simulink model "Charging"  (R2021a)
settings: Solver=VariableStepAuto  StartTime=0.0  StopTime=6000  RelTol=1e-3
undefined symbols (not defined in the file or in its folder): Ion, Lithium
libraries: spsBreakerLib x2, spsStairGeneratorLib x1, spsBatteryLib x1, simulink x1, spsControlledCurrentSourceLib x1, spsControlledVoltageSourceLib x1, spsVoltageMeasurementLib x1, spspowerguiLib x1
settings Model: Creator=Samiran  LastModifiedBy=Samiran

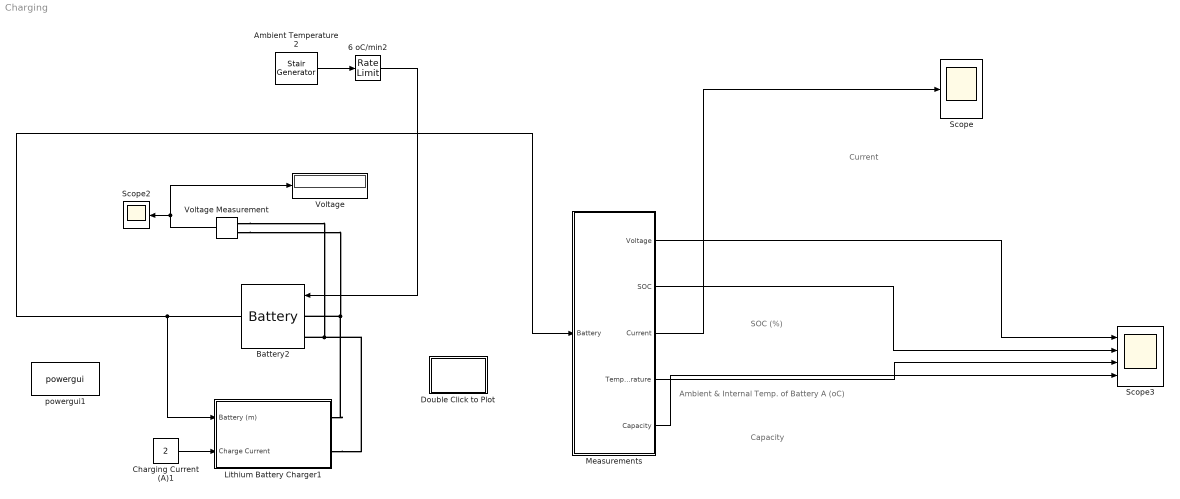
== system Charging ==
  note: Current
  note: Capacity
  note: SOC (%)
  note: Ambient & Internal Temp. of Battery A (oC)
  6 oC/min2 : RateLimiter  RisingSlewLimit=0.5  FallingSlewLimit=-0.5  SampleTimeMode=inherited
  Ambient Temperature2 : spsStairGeneratorLib/Stair Generator  t="[0, 500, 1000 1500  2000 2500 3000]"  e="[25, 0, -20  0  20, 50 20]"  Ts=0
  Battery2 : spsBatteryLib/Battery  BatType=Lithium-Ion  ShowTempParam=on  ThermalPreset="3.6V  3.6Ah  (LiNiO2)"  ShowAgeParam=on  NomV=3.1  NomQ=3.6  SOC=50  Batt_Tr=30  PresetModel=off  MaxQ=3.2  MinV=2.325  FullV=3.75  Dis_rate=0.72  R=0.00889  Normal_OP=2.8  expZone="[3.5         0.5]"  current=[6.5 13 32.5]  Units=Time  Tci=20  NomT=20  T2=0  MaxQ2=2.7  FullV2=3.5  Normal_OP2=2.94  expZone2="[3.25         0.5]"  Rca=0.6  ti=1000  Dp=0  Neq0=0  Tsim=1e6  Ta1=25  Qeol=5.4*0.9  Reol=0.013333*1.2  Char_age=[2.3478, 3]  Dis_age=[2.3478, 10]  N1=1500  N2=10500  N3=1000  N4=1400  Ta2=45  N5=950
  Charging Current (A)1 : Constant  Value=2
  Double Click to Plot : Subsystem
      settings: OpenFcn=LithiumBatteryChargingPlot
      mask Display: fprintf('Battery \n Charge Plot')
  Lithium Battery Charger1 : Subsystem  mask(Lithium Battery Charger){CV=4.2}
      mask prompts: CV "Saturation Charge Constant Voltage (V)"
      mask help:
      | Lithium Battery Charger Block Developed By Rodney Tan (PhD)
      | Version 1.00 (Aug 2019)
      |
      | This charger charge Lithium-Ion battery in two stages
      | This charger takes in charge current (A) from the input in (CC) Constant Current charging stage and switch to Saturation Charge (CV) Constant Voltage charging stage when the battery reaches the set constant voltage.
  Measurements : Subsystem
  Scope : Scope
  Scope2 : Scope
  Scope3 : Scope  NumInputPorts=4
  Voltage : Display
  Voltage Measurement : spsVoltageMeasurementLib/Voltage Measurement  PhasorSimulation=off  OutputType=Complex  PSBequivalent=0
  powergui1 : spspowerguiLib/powergui  Priority=1  SimulationMode=Continuous  SampleTime=50e-6  frequency=60  Iterations=50  frequencyindice=0  Pbase=100e6  ErrMax=1e-4  UnitsV=kV  UnitsW=MW  buscounter=0  FunctionMessages=off  echomessages=off  EnableUseOfTLC=off  CurrentSourceSwitches=off  DisableSnubberDevices=off  DisableRonSwitches=off  DisableVfSwitches=off  DisplayEquations=off  AutomaticDiscreteSolvers=off  SolverType=Tustin/Backward Euler (TBE)  Interpol=off  ExternalGateDelay=off  methode=off  Ts=100  x0status=blocks  SPID=on  SwTol=0  HookPort=off  NonlinearTolerance=1e-4  nMaxIteration=100  ContinueOnMaxIteration=off  RestoreLinks=warning  ResistiveCurrentMeasurement=off  Frange=[0:2:500]  Ylog=off  Xlog=on  ShowGrid=off  save=off  variable=ZData  structure=0  ZoomFFT=off  StartTime=0.0  cycles=1  DisplayStyle=1  fundamental=60  FreqAxis=off  MaxFrequency=1000  frequencyindicesteady=1  RmsSteady=1  display=off
  wires:
  Battery2/1 -> Lithium Battery Charger1/1(Battery (m)), Measurements/1("Battery ")
  6 oC/min2/1 -> Battery2/1
  Ambient Temperature2/1 -> 6 oC/min2/1
  Voltage Measurement/1 -> Voltage/1, Scope2/1
  Measurements/2(SOC) -> Scope3/2
  Charging Current (A)1/1 -> Lithium Battery Charger1/2(Charge Current)
  Measurements/4(Temperature) -> Scope3/3
  Measurements/5(Capacity) -> Scope3/4
  Measurements/1(Voltage) -> Scope3/1
  Measurements/3(Current) -> Scope/1
  connections:
  Voltage Measurement/LConn1 -- Lithium Battery Charger1/RConn1 -- Battery2/LConn1
  Voltage Measurement/LConn2 -- Battery2/LConn2 -- Lithium Battery Charger1/RConn2

== system Charging/Double Click to Plot ==

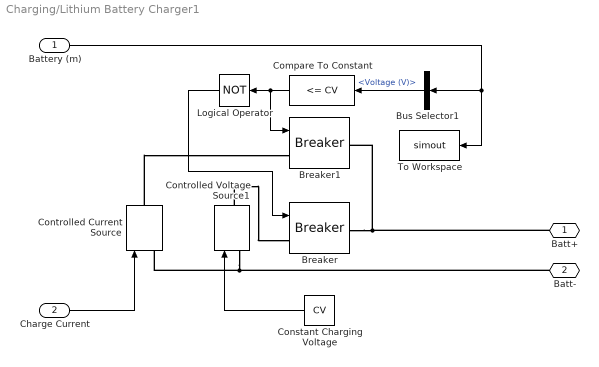
== system Charging/Lithium Battery Charger1 ==
  Battery (m) : Inport
  Charge Current : Inport  Port=2
  Breaker : spsBreakerLib/Breaker  InitialState=0  SwitchingTimes="[1/60  5/60]"  External=on  BreakerResistance=0.01  SnubberResistance=10e6  SnubberCapacitance=inf  Measurements=None  MoreParameters=on  NoBreakLoop=off
      settings: SourceProductBaseCode=PS
  Breaker1 : spsBreakerLib/Breaker  InitialState=0  SwitchingTimes="[1/60  5/60]"  External=on  BreakerResistance=0.01  SnubberResistance=1e6  SnubberCapacitance=inf  Measurements=None  MoreParameters=on  NoBreakLoop=off
      settings: SourceProductBaseCode=PS
  Bus Selector1 : BusSelector  OutputSignals=Voltage (V)
  Compare To Constant : simulink/Logic and Bit Operations/Compare To Constant  relop=<=  const=CV  OutDataTypeStr=boolean
  Constant Charging Voltage : Constant  Value=CV
  Controlled Current Source : spsControlledCurrentSourceLib/Controlled Current Source  Initialize=on  Source_Type=DC  Amplitude=0  Phase=0  Frequency=0  Measurements=None
  Controlled Voltage Source1 : spsControlledVoltageSourceLib/Controlled Voltage Source  Initialize=on  Source_Type=DC  Amplitude=0  Phase=0  Frequency=0  Measurements=None
  Logical Operator : Logic  Operator=NOT  AllPortsSameDT=off  OutDataTypeStr=boolean
  To Workspace : ToWorkspace  VariableName=simout  SampleTime=-1
  Batt+ : PMIOPort  Side=Right
  Batt- : PMIOPort  Port=2  Side=Right
  wires:
  Bus Selector1/1 -> Compare To Constant/1  "<Voltage (V)>"
  Constant Charging Voltage/1 -> Controlled Voltage Source1/1
  Battery (m)/1 -> To Workspace/1, Bus Selector1/1
  Logical Operator/1 -> Breaker/1
  Compare To Constant/1 -> Logical Operator/1, Breaker1/1
  Charge Current/1 -> Controlled Current Source/1
  connections:
  Breaker/RConn1 -- Batt+/RConn1 -- Breaker1/RConn1
  Controlled Voltage Source1/RConn1 -- Breaker/LConn1
  Controlled Current Source/RConn1 -- Breaker1/LConn1
  Controlled Voltage Source1/LConn1 -- Batt-/RConn1 -- Controlled Current Source/LConn1

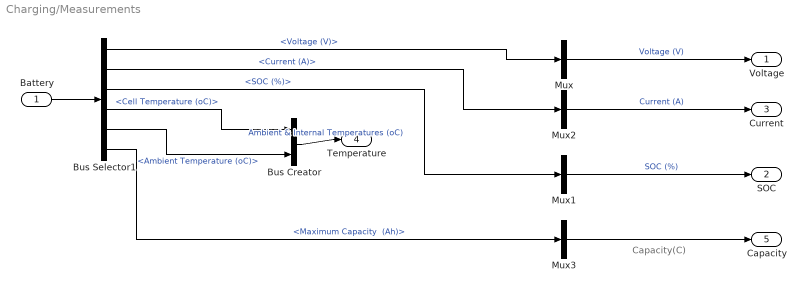
== system Charging/Measurements ==
  note: Capacity(C)
  "Battery " : Inport
  Bus Creator : BusCreator  Inputs=2
  Bus Selector1 : BusSelector  OutputSignals="Voltage (V),Current (A),SOC (%),Cell Temperature (oC),Ambient Temperature (oC),Maximum Capacity  (Ah)"
  Mux{,1..3} (4 alike) : Mux  Inputs=1
  Voltage : Outport  VectorParamsAs1DForOutWhenUnconnected=off
  SOC : Outport  Port=2  VectorParamsAs1DForOutWhenUnconnected=off
  Current : Outport  Port=3  VectorParamsAs1DForOutWhenUnconnected=off
  Temperature : Outport  Port=4  VectorParamsAs1DForOutWhenUnconnected=off
  Capacity : Outport  Port=5  VectorParamsAs1DForOutWhenUnconnected=off
  wires:
  Bus Selector1/4 -> Bus Creator/1  "<Cell Temperature (oC)>"
  Bus Selector1/5 -> Bus Creator/2  "<Ambient Temperature (oC)>"
  Bus Creator/1 -> Temperature/1  "Ambient & Internal Temperatures (oC)"
  Bus Selector1/3 -> Mux1/1  "<SOC (%)>"
  Mux1/1 -> SOC/1  "SOC (%)"
  Mux/1 -> Voltage/1  "Voltage (V)"
  Bus Selector1/1 -> Mux/1  "<Voltage (V)>"
  Bus Selector1/2 -> Mux2/1  "<Current (A)>"
  Mux2/1 -> Current/1  "Current (A)"
  "Battery "/1 -> Bus Selector1/1
  Bus Selector1/6 -> Mux3/1  "<Maximum Capacity  (Ah)>"
  Mux3/1 -> Capacity/1
